simulink model "lab2sim"  (R2023b)
settings: Solver=FixedStepAuto  StartTime=0.0  StopTime=stop_time  FixedStep=0.001  RelTol=1e-3
values from neighbouring files (symbols this model uses):
  a = 2    [lab2.m]
  a2 = 1    [lab2.m]
  a3 = 2    [lab2.m]
  B = 3    [lab2.m]
  B2 = 2    [lab2.m]
  b3 = 1    [lab2.m]
  B3 = 2    [lab2.m]
  e0 = e0w(i)    [lab2.m]
  e02 = e0w2(i)    [lab2.m]
  e03 = 1.5    [lab2.m]
  eprim0 = 0    [lab2.m]
  eprim02 = 0    [lab2.m]
  eprim03 = 0    [lab2.m]
  k = 3    [lab2.m]
  k2 = 2    [lab2.m]
  k3 = i    [lab2.m]
  T = 1    [lab2.m]
  T3 = 1    [lab2.m]
  w = 0    [lab2.m]
  w2 = 0    [lab2.m]
settings Model: Creator=pc  LastModifiedBy=pc

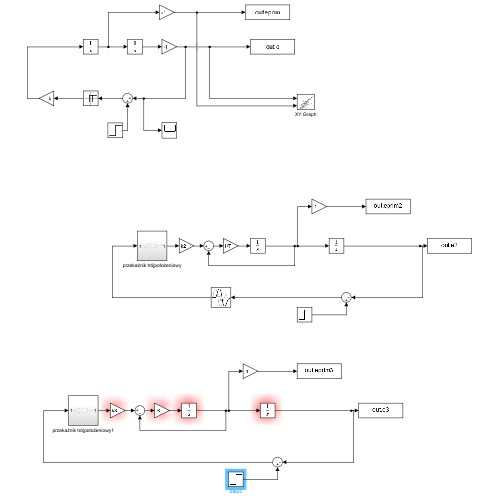
[thumbnail: Simulink's stored preview of the top-level diagram]
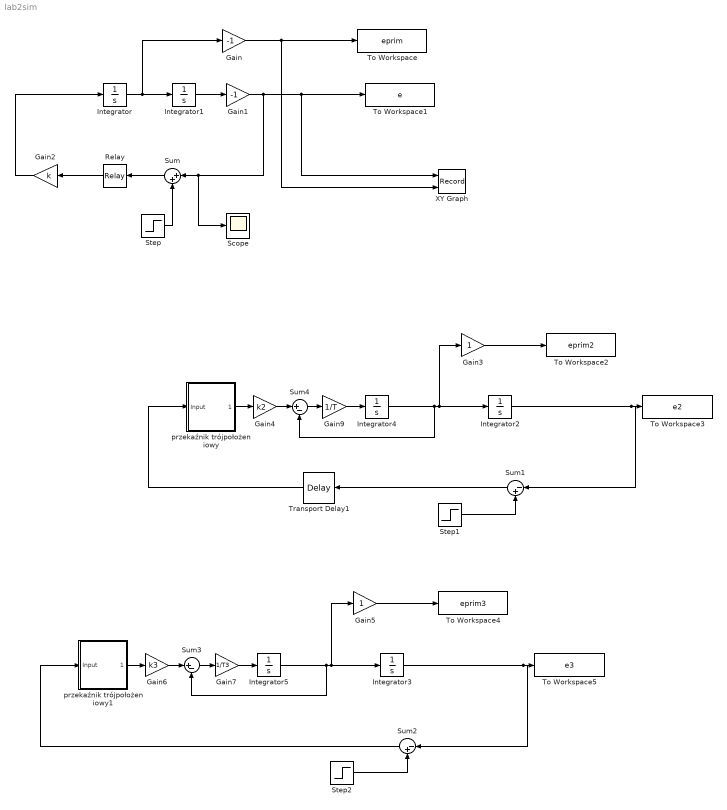
== system lab2sim ==
  Gain : Gain  Gain=-1
  Gain1 : Gain  Gain=-1
  Gain2 : Gain  Gain=k
  Gain3 : Gain
  Gain4 : Gain  Gain=k2
  Gain5 : Gain
  Gain6 : Gain  Gain=k3
  Gain7 : Gain  Gain=1/T3
  Gain9 : Gain  Gain=1/T
  Integrator : Integrator  InitialCondition=eprim0
  Integrator1 : Integrator  InitialCondition=e0
  Integrator2 : Integrator  InitialCondition=e02
  Integrator3 : Integrator  InitialCondition=e03
  Integrator4 : Integrator  InitialCondition=eprim02
  Integrator5 : Integrator  InitialCondition=eprim03
  Relay : Relay  OnSwitchValue=a  OffSwitchValue=-a  OnOutputValue=B  OffOutputValue=-B
  Scope : Scope
  Step : Step  Time=0  After=w  SampleTime=0
  Step1 : Step  Time=0  After=w2  SampleTime=0
  Step2 : Step  Time=0  After=0  SampleTime=0
  Sum : Sum  Inputs=|++
  Sum1 : Sum  Inputs=|-+
  Sum2 : Sum  Inputs=|-+
  Sum3 : Sum  Inputs=|+-
  Sum4 : Sum  Inputs=|+-
  To Workspace : ToWorkspace  VariableName=eprim  SaveFormat=Timeseries  SampleTime=-1
  To Workspace1 : ToWorkspace  VariableName=e  SaveFormat=Timeseries  SampleTime=-1
  To Workspace2 : ToWorkspace  VariableName=eprim2  SaveFormat=Timeseries  SampleTime=-1
  To Workspace3 : ToWorkspace  VariableName=e2  SaveFormat=Timeseries  SampleTime=-1
  To Workspace4 : ToWorkspace  VariableName=eprim3  SaveFormat=Timeseries  SampleTime=-1
  To Workspace5 : ToWorkspace  VariableName=e3  SaveFormat=Timeseries  SampleTime=-1
  Transport Delay1 : TransportDelay
  XY Graph : Record  FileSettingsInternal="{\"entries\":[{\"content\":{\"excelSettings\":{\"content\":{},\"type\":\"Streamout.ExcelSettings\"}},\"type\":\"Streamout.FileSettingStorage\",\"uuid\":\"\"}],\"packageUris\":[\"http:\\/\\/schema.mathworks.com\\/mf0\\/streamout_blocks\\/R2020a\"],\"version\":\"1.0\"}"  Layout=[1 1]  SignalsInternal="{\"entries\":[{\"content\":{\"signals\":[{\"content\":{\"blockPath\":[],\"dimensions\":[1],\"domain\":\"\",\"lineColor\":\"#a2142f\",\"plots\":[ 1 ],\"port\":1,\"sid\":[\"\"],\"signalID\":1,\"signalName\":\"Gain1\"},\"type\":\"RecordBlkView.Signal\",\"uuid\":\"\"},{\"content\":{\"blockPath\":[],\"dimensions\":[1],\"domain\":\"\",\"lineColor\":\"#139fff\",\"plots\":[ 1 ],\"port\":2,\"sid\":[\"\"],\"signalID\":2,\"signalName\":\"Gain\"},\"type\":\"RecordBlkView.Signal\",\"uuid\":\"\"}]},\"type\":\"RecordBlkView.InputSignals\",\"uuid\":\"\"}],\"packageUris\":[\"http:\\/\\/schema.mathworks.com\\/mf0\\/streamout_blocks\\/R2020a\"],\"version\":\"1.0\"}"  VisualizationBindings="{\"xyplotplugin\":{\"info\":[{\"series\":[{\"bindingParametersList\":[{\"parameter\":\"X-Axis\",\"signalID\":1,\"signalName\":\"Gain1\"},{\"parameter\":\"Y-Axis\",\"signalID\":2,\"signalName\":\"Gain\"}],\"seriesID\":0}],\"subplotID\":1}]}}"  CompatibilityTag=XY
  przekaźnik trójpołożeniowy : Subsystem
  przekaźnik trójpołożeniowy1 : Subsystem
  wires:
  Integrator/1 -> Gain/1, Integrator1/1
  Gain/1 -> XY Graph/2, To Workspace/1
  Integrator1/1 -> Gain1/1
  Gain1/1 -> Sum/1, Scope/1, XY Graph/1, To Workspace1/1
  Relay/1 -> Gain2/1
  Gain2/1 -> Integrator/1
  Sum/1 -> Relay/1
  Step/1 -> Sum/2
  Gain3/1 -> To Workspace2/1
  Step1/1 -> Sum1/2
  Integrator4/1 -> Sum4/2, Integrator2/1, Gain3/1
  przekaźnik trójpołożeniowy/1(Output) -> Gain4/1
  Gain4/1 -> Sum4/1
  Sum4/1 -> Gain9/1
  Gain9/1 -> Integrator4/1
  Integrator2/1 -> Sum1/1, To Workspace3/1
  Sum1/1 -> Transport Delay1/1
  Transport Delay1/1 -> przekaźnik trójpołożeniowy/1(Input)
  przekaźnik trójpołożeniowy1/1(Output) -> Gain6/1
  Sum3/1 -> Gain7/1
  Gain7/1 -> Integrator5/1
  Integrator3/1 -> Sum2/1, To Workspace5/1
  Gain6/1 -> Sum3/1
  Integrator5/1 -> Sum3/2, Integrator3/1, Gain5/1
  Step2/1 -> Sum2/2
  Sum2/1 -> przekaźnik trójpołożeniowy1/1(Input)
  Gain5/1 -> To Workspace4/1

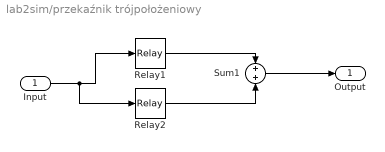
== system lab2sim/przekaźnik trójpołożeniowy ==
  Input : Inport
  Relay1 : Relay  OnSwitchValue=a2  OffSwitchValue=a2  OnOutputValue=B2
  Relay2 : Relay  OnSwitchValue=-a2  OffSwitchValue=-a2  OnOutputValue=0  OffOutputValue=-B2
  Sum1 : Sum  Inputs=+|+
  Output : Outport
  wires:
  Input/1 -> Relay2/1, Relay1/1
  Relay2/1 -> Sum1/2
  Sum1/1 -> Output/1
  Relay1/1 -> Sum1/1

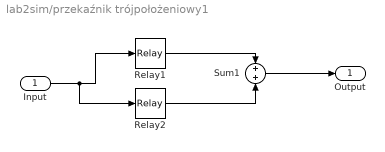
== system lab2sim/przekaźnik trójpołożeniowy1 ==
  Input : Inport
  Relay1 : Relay  OnSwitchValue=a3  OffSwitchValue=b3  OnOutputValue=B3
  Relay2 : Relay  OnSwitchValue=-b3  OffSwitchValue=-a3  OnOutputValue=0  OffOutputValue=-B3
  Sum1 : Sum  Inputs=+|+
  Output : Outport
  wires:
  Input/1 -> Relay2/1, Relay1/1
  Relay2/1 -> Sum1/2
  Sum1/1 -> Output/1
  Relay1/1 -> Sum1/1
